simulink model "model"  (R2018b)
settings: Solver=FixedStepAuto  StartTime=0.0  StopTime=sim_time  FixedStep=Ts/10  RelTol=1e-3
StopFcn:
  | %figure;plot(true_position.Data(:,1),true_position.Data(:,2))
values from neighbouring files (symbols this model uses):
  b = ((W*a - F4*l)*cos(theta)) / (W*sin(theta)),    [blackbike_CoM.m]    (also in main.m = 1.15)
  bike_params = [g h b a lambda m]    [main.m]
  D_balancing = kd_vec(i)    [bike_linear_analysis_balancing.m]    (also in main.m = 0.01)
  D_heading = 0.01    [main.m]
  D_lateral = 0.01    [main.m]
  delay_steering = 4    [main.m]
  den_tf_steering = [1 50]    [main.m]
  g = 9.81    [main.m]
  heading_control = 0    [main.m]
  I_balancing = 0    [main.m]
  I_heading = -0.01    [main.m]
  I_lateral = 0    [main.m]
  IMU_height = 0.215    [main.m]
  initial_roll = deg2rad(2)    [main.m]
  initial_rollrate = deg2rad(1)    [main.m]
  initial_x = 0    [main.m]
  initial_y = 0    [main.m]
  lambda = deg2rad(90-24)    [main.m]
  lateral_control = 0    [main.m]
  num_tf_steering = [50]    [main.m]
  P_balancing = 1    [bike_linear_analysis_balancing.m]    (also in main.m)
  P_heading = -0.1    [main.m]
  P_lateral = -0.07    [main.m]
  path_tracking = 0    [main.m]
  path_x = path_x'    [paths.m]
  path_y = path_y'    [paths.m]
  Ts = 0.01    [main.m]
  v = 14/3.6    (= 3.88888888889)    [main.m]
undefined symbols (not defined in the file or in its folder): A, B, C, cumulative_dist_along_path, D
libraries: simulink x9, simulink_extras x7, dspsigops x2
settings Model: Creator=maximef  LastModifiedBy=maximef

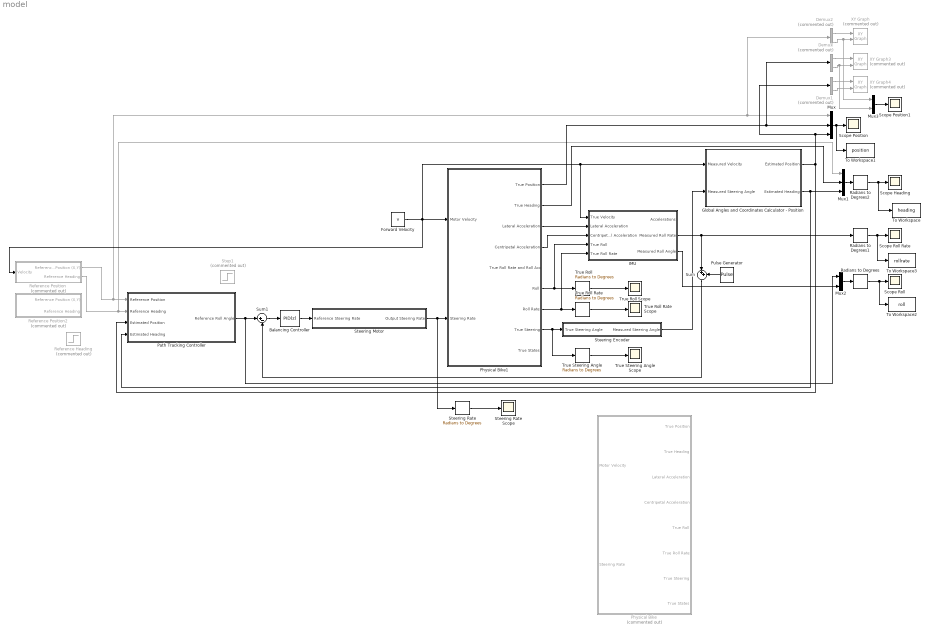
== system model ==
  Balancing Controller : simulink/Continuous/PID Controller  Controller=PID  Form=Ideal  TimeDomain=Discrete-time  SampleTime=Ts  IntegratorMethod=Trapezoidal  FilterMethod=Forward Euler  ControllerParametersSource=internal  P=P_balancing  I=I_balancing  D=D_balancing  UseFilter=off  N=5  TunerSelectOption=Transfer Function Based (PID Tuner App)  InitialConditionSource=internal  InitialConditionForIntegrator=0  InitialConditionForFilter=0  DifferentiatorICPrevScaledInput=0  ExternalReset=none  TrackingMode=off  Kt=1  LimitOutput=off  UpperSaturationLimit=inf  LowerSaturationLimit=-inf  LinearizeAsGain=on  AntiWindupMode=none  Kb=1  POutMin=[]  POutMax=[]  IOutMin=[]  IOutMax=[]  DOutMin=[]  DOutMax=[]  NOutMin=[]  NOutMax=[]  SumOutMin=[]  SumOutMax=[]  SaturationOutMin=[]  SaturationOutMax=[]  PParamMin=[]  PParamMax=[]  IParamMin=[]  IParamMax=[]  DParamMin=[]  DParamMax=[]  NParamMin=[]  NParamMax=[]  KbParamMin=[]  KbParamMax=[]  KtParamMin=[]  KtParamMax=[]  KbOutMin=[]  KbOutMax=[]  KtOutMin=[]  KtOutMax=[]  IntegratorOutMin=[]  IntegratorOutMax=[]  FilterOutMin=[]  FilterOutMax=[]  SumI1OutMin=[]  SumI1OutMax=[]  SumI2OutMin=[]  SumI2OutMax=[]  SumI3OutMin=[]  SumI3OutMax=[]  SumI4OutMin=[]  SumI4OutMax=[]  SumDOutMin=[]  SumDOutMax=[]  DifferentiatorOutMin=[]  DifferentiatorOutMax=[]  FilterDiffOutCoefMin=[]  FilterDiffOutCoefMax=[]  ReciprocalOutMin=[]  ReciprocalOutMax=[]  SumDenOutMin=[]  SumDenOutMax=[]  SumNumOutMin=[]  SumNumOutMax=[]  DivideOutMin=[]  DivideOutMax=[]  IntegratorContinuousStateAttributes=''  IntegratorStateMustResolveToSignalObject=off  IntegratorRTWStateStorageClass=Auto  FilterContinuousStateAttributes=''  FilterStateMustResolveToSignalObject=off  FilterRTWStateStorageClass=Auto  ParallelPVariant=Passthrough  IdealPVariant=InternalParameters  IVariant=InternalParameters  DVariant=InternalParameters  IntegratorVariant=Discrete  SatVariant=Disabled  AWVariant=Passthrough  PCopyVariant=Disabled  TRVariant=Disabled  FdbkBlocksVariant=Forward  IdealPFdbkVariant=Disabled  SatFdbkVariant=Disabled  DerivativeFilterVariant=Differentiator  NVariant=Passthrough  NCopyVariant=Disabled_SignalSpec  FilterICVariant=InternalICsDifferentiator  IntegratorICVariant=InternalICs  ExternalResetVariant=Disabled  TRSumVariant=Passthrough  SumFdbkVariant=Disabled  SumVariant=Sum_PID
  Demux : Demux  Commented=on  Outputs=2
  Demux1 : Demux  Commented=on  Outputs=2
  Demux2 : Demux  Commented=on  Outputs=2
  Forward Velocity : Constant  Value=v
  Global Angles and Coordinates Calculator - Position : Subsystem  SystemSampleTime=Ts
  IMU : Subsystem  TreatAsAtomicUnit=on
  Mux : Mux  Inputs=3
  Mux1 : Mux  Inputs=3
  Mux2 : Mux  Inputs=2
  Mux3 : Mux  Inputs=2
  Path Tracking Controller : Subsystem
  Physical Bike : Subsystem  Commented=on
  Physical Bike1 : Subsystem
  Pulse Generator : DiscretePulseGenerator  PulseType=Time based  Amplitude=deg2rad(1)  Period=10  PulseWidth=10
  Radians to Degrees : simulink_extras/Transformations/Radians to Degrees
  Radians to Degrees1 : simulink_extras/Transformations/Radians to Degrees
  Radians to Degrees2 : simulink_extras/Transformations/Radians to Degrees
  Reference Heading : Step  Commented=on  SampleTime=0
  Reference Position : Subsystem  Commented=on
  Reference Position2 : Subsystem  Commented=on
  Scope Heading : Scope
  Scope Position : Scope
  Scope Position1 : Scope
  Scope Roll : Scope
  Scope Roll Rate : Scope
  Steering Encoder : Subsystem  TreatAsAtomicUnit=on  SystemSampleTime=Ts
  Steering Motor : Subsystem
  Steering Rate : simulink_extras/Transformations/Radians to Degrees
  Steering Rate Scope : Scope
  Step1 : Step  Commented=on  Time=0  After=0  SampleTime=0
  Sum : Sum  Inputs=|++
  Sum1 : Sum  Inputs=|+-
  To Workspace : ToWorkspace  VariableName=heading  SaveFormat=Timeseries  SampleTime=-1
  To Workspace1 : ToWorkspace  VariableName=position  SaveFormat=Timeseries  SampleTime=-1
  To Workspace2 : ToWorkspace  VariableName=roll  SaveFormat=Timeseries  SampleTime=-1
  To Workspace3 : ToWorkspace  VariableName=rollrate  SaveFormat=Timeseries  SampleTime=-1
  True Roll : simulink_extras/Transformations/Radians to Degrees
  True Roll Rate : simulink_extras/Transformations/Radians to Degrees
  True Roll Rate Scope : Scope
  True Roll Scope : Scope
  True Steering Angle : simulink_extras/Transformations/Radians to Degrees
  True Steering Angle Scope : Scope
  XY Graph : simulink/Sinks/XY Graph  Commented=on  xmin=-10  xmax=100  ymin=-1  ymax=1  st=-1
  XY Graph3 : simulink/Sinks/XY Graph  Commented=on  xmin=-50  xmax=50  ymin=-50  ymax=50  st=-1
  XY Graph4 : simulink/Sinks/XY Graph  Commented=on  xmin=-50  xmax=50  ymin=-50  ymax=50  st=-1
  wires:
  True Roll Rate/1 -> True Roll Rate Scope/1
  True Steering Angle/1 -> True Steering Angle Scope/1
  True Roll/1 -> True Roll Scope/1
  Physical Bike1/8(True Steering) -> True Steering Angle/1, Steering Encoder/1(True Steering Angle)
  Physical Bike1/7(Roll Rate) -> IMU/5(True Roll Rate), True Roll Rate/1
  Sum1/1 -> Balancing Controller/1
  Reference Position/1(Reference Position (X,Y)) -> Demux2/1, Mux/1, Path Tracking Controller/1(Reference Position)
  Reference Position/2(Reference Heading) -> Mux1/1, Path Tracking Controller/2(Reference Heading)
  Physical Bike1/6(Roll) -> IMU/4(True Roll), True Roll/1
  Physical Bike1/2(True Heading) -> Mux1/2
  Physical Bike1/4(Centripetal Acceleration) -> IMU/3(Centripetal Acceleration)
  Forward Velocity/1 -> Reference Position/1(Velocity), Physical Bike1/1(Motor Velocity), IMU/1(True Velocity), Global Angles and Coordinates Calculator - Position/1(Measured Velocity)
  Steering Encoder/1(Measured Steering Angle) -> Global Angles and Coordinates Calculator - Position/2(Measured Steering Angle)
  Global Angles and Coordinates Calculator - Position/1(Estimated Position) -> Mux/3, Demux1/1, Path Tracking Controller/3(Estimated Position)
  Global Angles and Coordinates Calculator - Position/2(Estimated Heading) -> Path Tracking Controller/4(Estimated Heading), Mux1/3
  Mux/1 -> To Workspace1/1, Scope Position/1
  Physical Bike1/1(True Position) -> Demux/1, Mux/2
  Mux1/1 -> Radians to Degrees2/1
  IMU/3(Measured Roll Angle) -> Mux2/2
  Mux2/1 -> Radians to Degrees/1
  Path Tracking Controller/1(Reference Roll Angle) -> Sum1/1, Mux2/1
  IMU/2(Measured Roll Rate) -> Sum/1, Radians to Degrees1/1
  Radians to Degrees/1 -> To Workspace2/1, Scope Roll/1
  Radians to Degrees1/1 -> To Workspace3/1, Scope Roll Rate/1
  Radians to Degrees2/1 -> To Workspace/1, Scope Heading/1
  Demux2/1 -> XY Graph/1
  Demux/1 -> XY Graph3/1
  Demux2/2 -> Mux3/1, XY Graph/2
  Demux/2 -> Mux3/2, XY Graph3/2
  Demux1/2 -> XY Graph4/2
  Demux1/1 -> XY Graph4/1
  Mux3/1 -> Scope Position1/1
  Physical Bike1/3(Lateral Acceleration) -> IMU/2(Lateral Acceleration)
  Steering Rate/1 -> Steering Rate Scope/1
  Sum/1 -> Sum1/2
  Balancing Controller/1 -> Steering Motor/1(Reference Steering Rate)
  Steering Motor/1(Output Steering Rate) -> Physical Bike1/2(Steering Rate), Steering Rate/1
  Pulse Generator/1 -> Sum/2

== system model/Global Angles and Coordinates Calculator - Position ==
  Measured Velocity : Inport
  Measured Steering Angle : Inport  Port=2
  Gain1 : Gain  Gain=sin(lambda)
  Measured Bike Angles to Global Angles : Subsystem
  Measured Global Angles to Global Coordinates : Subsystem
  Sum : Sum  Inputs=++|
  Estimated Position : Outport
  Estimated Heading : Outport  Port=2
  wires:
  Measured Bike Angles to Global Angles/1(Psi) -> Sum/2, Measured Global Angles to Global Coordinates/2(Psi)
  Gain1/1 -> Measured Bike Angles to Global Angles/2(Measured Steering Angle)
  Sum/1 -> Estimated Heading/1
  Measured Bike Angles to Global Angles/2(Beta) -> Sum/1, Measured Global Angles to Global Coordinates/3(Beta)
  Measured Global Angles to Global Coordinates/1("Position (X, Y)") -> Estimated Position/1
  Measured Velocity/1 -> Measured Global Angles to Global Coordinates/1(Velocity), Measured Bike Angles to Global Angles/1(Velocity)
  Measured Steering Angle/1 -> Gain1/1

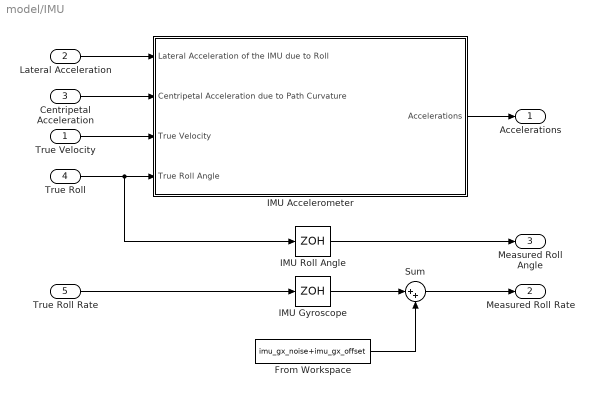
== system model/IMU ==
  True Velocity : Inport
  Lateral Acceleration : Inport  Port=2
  Centripetal Acceleration : Inport  Port=3
  True Roll : Inport  Port=4
  True Roll Rate : Inport  Port=5
  From Workspace : FromWorkspace  VariableName=imu_gx_noise+imu_gx_offset  SampleTime=0
  IMU Accelerometer : Subsystem
  IMU Gyroscope : ZeroOrderHold  SampleTime=Ts
  IMU Roll Angle : ZeroOrderHold  SampleTime=Ts
  Sum : Sum  Inputs=|++
  Accelerations : Outport
  Measured Roll Rate : Outport  Port=2
  Measured Roll Angle : Outport  Port=3
  wires:
  True Velocity/1 -> IMU Accelerometer/3(True Velocity)
  Lateral Acceleration/1 -> IMU Accelerometer/1(Lateral Acceleration of the IMU due to Roll)
  Centripetal Acceleration/1 -> IMU Accelerometer/2(Centripetal Acceleration due to Path Curvature)
  True Roll/1 -> IMU Roll Angle/1, IMU Accelerometer/4(True Roll Angle)
  IMU Accelerometer/1(Accelerations) -> Accelerations/1
  IMU Gyroscope/1 -> Sum/1
  True Roll Rate/1 -> IMU Gyroscope/1
  IMU Roll Angle/1 -> Measured Roll Angle/1
  Sum/1 -> Measured Roll Rate/1
  From Workspace/1 -> Sum/2

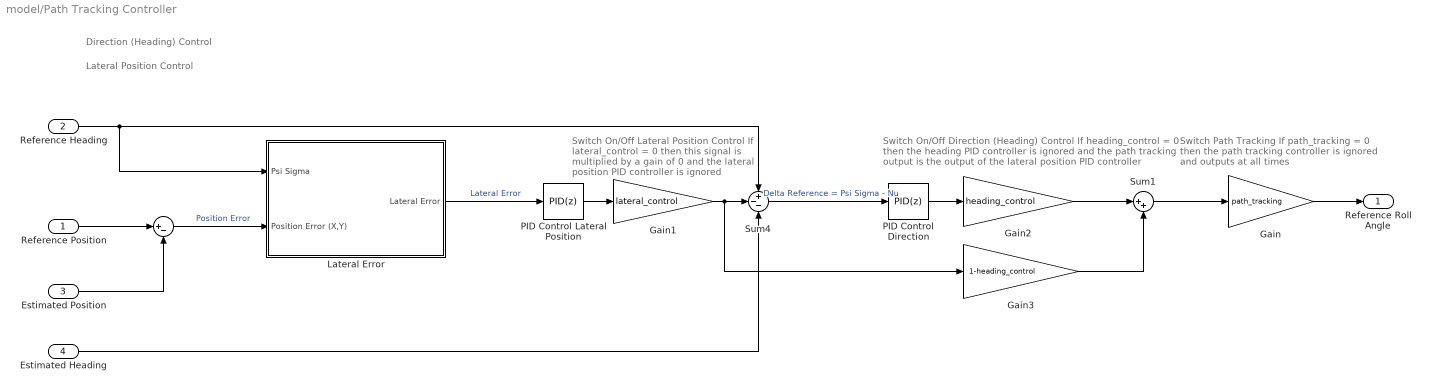
== system model/Path Tracking Controller ==
  note: Direction (Heading) Control
  note: Lateral Position Control
  note: Switch On/Off Lateral Position Control
      | If lateral_control = 0 then this signal
      | is multiplied by a gain of 0 and the
      | lateral position PID controller is ignored
  note: Switch Path Tracking
      | If path_tracking = 0 then the path tracking controller
      | is ignored and outputs at all times
  note: Switch On/Off Direction (Heading) Control
      | If heading_control = 0 then the heading PID controller is ignored
      | and the path tracking output is the output of the lateral position PID controller
  Reference Position : Inport
  Reference Heading : Inport  Port=2
  Estimated Position : Inport  Port=3
  Estimated Heading : Inport  Port=4
  " " : Sum  Inputs=|+-
  Gain : Gain  Gain=path_tracking
  Gain1 : Gain  Gain=lateral_control
  Gain2 : Gain  Gain=heading_control
  Gain3 : Gain  Gain=1-heading_control
  Lateral Error : Subsystem  SystemSampleTime=Ts
  PID Control Lateral Position : simulink/Continuous/PID Controller  Controller=PID  Form=Parallel  TimeDomain=Discrete-time  SampleTime=Ts  IntegratorMethod=Forward Euler  FilterMethod=Forward Euler  ControllerParametersSource=internal  P=P_lateral  I=I_lateral  D=D_lateral  UseFilter=on  N=100  TunerSelectOption=Transfer Function Based (PID Tuner App)  InitialConditionSource=internal  InitialConditionForIntegrator=0  InitialConditionForFilter=0  DifferentiatorICPrevScaledInput=0  ExternalReset=none  TrackingMode=off  Kt=1  LimitOutput=off  UpperSaturationLimit=inf  LowerSaturationLimit=-inf  LinearizeAsGain=on  AntiWindupMode=none  Kb=1  POutMin=[]  POutMax=[]  IOutMin=[]  IOutMax=[]  DOutMin=[]  DOutMax=[]  NOutMin=[]  NOutMax=[]  SumOutMin=[]  SumOutMax=[]  SaturationOutMin=[]  SaturationOutMax=[]  PParamMin=[]  PParamMax=[]  IParamMin=[]  IParamMax=[]  DParamMin=[]  DParamMax=[]  NParamMin=[]  NParamMax=[]  KbParamMin=[]  KbParamMax=[]  KtParamMin=[]  KtParamMax=[]  KbOutMin=[]  KbOutMax=[]  KtOutMin=[]  KtOutMax=[]  IntegratorOutMin=[]  IntegratorOutMax=[]  FilterOutMin=[]  FilterOutMax=[]  SumI1OutMin=[]  SumI1OutMax=[]  SumI2OutMin=[]  SumI2OutMax=[]  SumI3OutMin=[]  SumI3OutMax=[]  SumI4OutMin=[]  SumI4OutMax=[]  SumDOutMin=[]  SumDOutMax=[]  DifferentiatorOutMin=[]  DifferentiatorOutMax=[]  FilterDiffOutCoefMin=[]  FilterDiffOutCoefMax=[]  ReciprocalOutMin=[]  ReciprocalOutMax=[]  SumDenOutMin=[]  SumDenOutMax=[]  SumNumOutMin=[]  SumNumOutMax=[]  DivideOutMin=[]  DivideOutMax=[]  IntegratorContinuousStateAttributes=''  IntegratorStateMustResolveToSignalObject=off  IntegratorRTWStateStorageClass=Auto  FilterContinuousStateAttributes=''  FilterStateMustResolveToSignalObject=off  FilterRTWStateStorageClass=Auto  ParallelPVariant=InternalParameters  IdealPVariant=Disabled  IVariant=InternalParameters  DVariant=InternalParameters  IntegratorVariant=Discrete  SatVariant=Disabled  AWVariant=Passthrough  PCopyVariant=Disabled  TRVariant=Disabled  FdbkBlocksVariant=Forward  IdealPFdbkVariant=Disabled  SatFdbkVariant=Disabled  DerivativeFilterVariant=ForwardEulerFilter  NVariant=InternalParameters  NCopyVariant=Disabled  FilterICVariant=InternalICsFilter  IntegratorICVariant=InternalICs  ExternalResetVariant=Disabled  TRSumVariant=Passthrough  SumFdbkVariant=Disabled  SumVariant=Sum_PID
  PID Control Direction : simulink/Continuous/PID Controller  Controller=PID  Form=Parallel  TimeDomain=Discrete-time  SampleTime=Ts  IntegratorMethod=Forward Euler  FilterMethod=Forward Euler  ControllerParametersSource=internal  P=P_heading  I=I_heading  D=D_heading  UseFilter=on  N=100  TunerSelectOption=Transfer Function Based (PID Tuner App)  InitialConditionSource=internal  InitialConditionForIntegrator=0  InitialConditionForFilter=0  DifferentiatorICPrevScaledInput=0  ExternalReset=none  TrackingMode=off  Kt=1  LimitOutput=off  UpperSaturationLimit=inf  LowerSaturationLimit=-inf  LinearizeAsGain=on  AntiWindupMode=none  Kb=1  POutMin=[]  POutMax=[]  IOutMin=[]  IOutMax=[]  DOutMin=[]  DOutMax=[]  NOutMin=[]  NOutMax=[]  SumOutMin=[]  SumOutMax=[]  SaturationOutMin=[]  SaturationOutMax=[]  PParamMin=[]  PParamMax=[]  IParamMin=[]  IParamMax=[]  DParamMin=[]  DParamMax=[]  NParamMin=[]  NParamMax=[]  KbParamMin=[]  KbParamMax=[]  KtParamMin=[]  KtParamMax=[]  KbOutMin=[]  KbOutMax=[]  KtOutMin=[]  KtOutMax=[]  IntegratorOutMin=[]  IntegratorOutMax=[]  FilterOutMin=[]  FilterOutMax=[]  SumI1OutMin=[]  SumI1OutMax=[]  SumI2OutMin=[]  SumI2OutMax=[]  SumI3OutMin=[]  SumI3OutMax=[]  SumI4OutMin=[]  SumI4OutMax=[]  SumDOutMin=[]  SumDOutMax=[]  DifferentiatorOutMin=[]  DifferentiatorOutMax=[]  FilterDiffOutCoefMin=[]  FilterDiffOutCoefMax=[]  ReciprocalOutMin=[]  ReciprocalOutMax=[]  SumDenOutMin=[]  SumDenOutMax=[]  SumNumOutMin=[]  SumNumOutMax=[]  DivideOutMin=[]  DivideOutMax=[]  IntegratorContinuousStateAttributes=''  IntegratorStateMustResolveToSignalObject=off  IntegratorRTWStateStorageClass=Auto  FilterContinuousStateAttributes=''  FilterStateMustResolveToSignalObject=off  FilterRTWStateStorageClass=Auto  ParallelPVariant=InternalParameters  IdealPVariant=Disabled  IVariant=InternalParameters  DVariant=InternalParameters  IntegratorVariant=Discrete  SatVariant=Disabled  AWVariant=Passthrough  PCopyVariant=Disabled  TRVariant=Disabled  FdbkBlocksVariant=Forward  IdealPFdbkVariant=Disabled  SatFdbkVariant=Disabled  DerivativeFilterVariant=ForwardEulerFilter  NVariant=InternalParameters  NCopyVariant=Disabled  FilterICVariant=InternalICsFilter  IntegratorICVariant=InternalICs  ExternalResetVariant=Disabled  TRSumVariant=Passthrough  SumFdbkVariant=Disabled  SumVariant=Sum_PID
  Sum1 : Sum  Inputs=|++
  Sum4 : Sum  Inputs=+--
  Reference Roll Angle : Outport
  wires:
  Lateral Error/1(Lateral Error) -> PID Control Lateral Position/1  "Lateral Error"
  Estimated Position/1 -> " "/2
  " "/1 -> Lateral Error/2(Position Error (X,Y))  "Position Error"
  Sum4/1 -> PID Control Direction/1  "Delta Reference = Psi Sigma - Nu"
  Estimated Heading/1 -> Sum4/3
  Gain1/1 -> Sum4/2, Gain3/1
  PID Control Lateral Position/1 -> Gain1/1
  Reference Heading/1 -> Sum4/1, Lateral Error/1(Psi Sigma)
  Reference Position/1 -> " "/1
  Gain2/1 -> Sum1/1
  Gain3/1 -> Sum1/2
  Sum1/1 -> Gain/1
  Gain/1 -> Reference Roll Angle/1
  PID Control Direction/1 -> Gain2/1

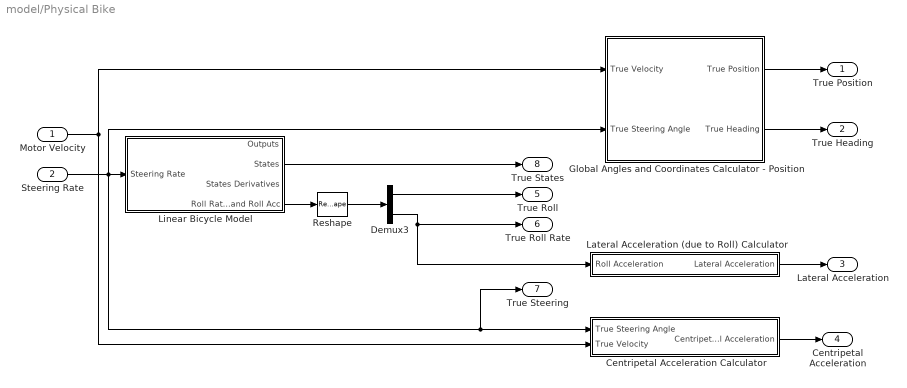
== system model/Physical Bike ==
  Motor Velocity : Inport
  Steering Rate : Inport  Port=2
  Centripetal Acceleration Calculator : Subsystem
  Demux3 : Demux  Outputs=2
  Global Angles and Coordinates Calculator - Position : Subsystem  SystemSampleTime=Ts
  Lateral Acceleration (due to Roll) Calculator : Subsystem
  Linear Bicycle Model : Subsystem
  Reshape : Reshape
  True Position : Outport
  True Heading : Outport  Port=2
  Lateral Acceleration : Outport  Port=3
  Centripetal Acceleration : Outport  Port=4
  True Roll : Outport  Port=5
  True Roll Rate : Outport  Port=6
  True Steering : Outport  Port=7
  True States : Outport  Port=8
  wires:
  Steering Rate/1 -> Global Angles and Coordinates Calculator - Position/2(True Steering Angle), True Steering/1, Centripetal Acceleration Calculator/1(True Steering Angle), Linear Bicycle Model/1(Steering Rate)
  Centripetal Acceleration Calculator/1(Centripetal Acceleration) -> Centripetal Acceleration/1
  Demux3/2 -> True Roll Rate/1, Lateral Acceleration (due to Roll) Calculator/1(Roll Acceleration)
  Lateral Acceleration (due to Roll) Calculator/1(Lateral Acceleration) -> Lateral Acceleration/1
  Linear Bicycle Model/2(States) -> True States/1
  Reshape/1 -> Demux3/1
  Linear Bicycle Model/4(Roll Rate and Roll Acc) -> Reshape/1
  Motor Velocity/1 -> Centripetal Acceleration Calculator/2(True Velocity), Global Angles and Coordinates Calculator - Position/1(True Velocity)
  Global Angles and Coordinates Calculator - Position/1(True Position) -> True Position/1
  Global Angles and Coordinates Calculator - Position/2(True Heading) -> True Heading/1
  Demux3/1 -> True Roll/1

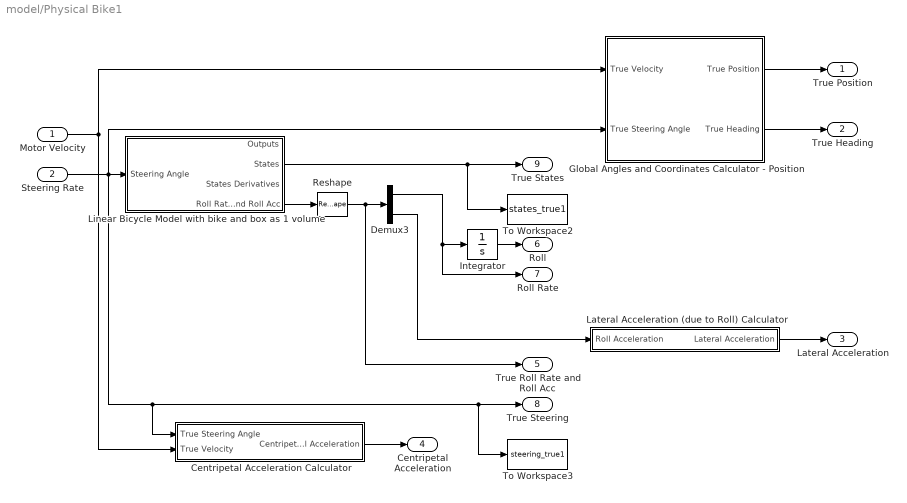
== system model/Physical Bike1 ==
  Motor Velocity : Inport
  Steering Rate : Inport  Port=2
  Centripetal Acceleration Calculator : Subsystem
  Demux3 : Demux  Outputs=2
  Global Angles and Coordinates Calculator - Position : Subsystem  SystemSampleTime=Ts
  Integrator : Integrator  InitialCondition=initial_roll
  Lateral Acceleration (due to Roll) Calculator : Subsystem
  Linear Bicycle Model with bike and box as 1 volume : Subsystem
  Reshape : Reshape
  To Workspace2 : ToWorkspace  VariableName=states_true1  SaveFormat=Timeseries  SampleTime=-1
  To Workspace3 : ToWorkspace  VariableName=steering_true1  SaveFormat=Timeseries  SampleTime=-1
  True Position : Outport
  True Heading : Outport  Port=2
  Lateral Acceleration : Outport  Port=3
  Centripetal Acceleration : Outport  Port=4
  True Roll Rate and Roll Acc : Outport  Port=5
  Roll : Outport  Port=6
  Roll Rate : Outport  Port=7
  True Steering : Outport  Port=8
  True States : Outport  Port=9
  wires:
  Steering Rate/1 -> Global Angles and Coordinates Calculator - Position/2(True Steering Angle), To Workspace3/1, True Steering/1, Centripetal Acceleration Calculator/1(True Steering Angle), Linear Bicycle Model with bike and box as 1 volume/1(Steering Angle)
  Centripetal Acceleration Calculator/1(Centripetal Acceleration) -> Centripetal Acceleration/1
  Demux3/2 -> Lateral Acceleration (due to Roll) Calculator/1(Roll Acceleration)
  Lateral Acceleration (due to Roll) Calculator/1(Lateral Acceleration) -> Lateral Acceleration/1
  Linear Bicycle Model with bike and box as 1 volume/2(States) -> To Workspace2/1, True States/1
  Demux3/1 -> Integrator/1, Roll Rate/1
  Reshape/1 -> True Roll Rate and Roll Acc/1, Demux3/1
  Linear Bicycle Model with bike and box as 1 volume/4(Roll Rate and Roll Acc) -> Reshape/1
  Motor Velocity/1 -> Centripetal Acceleration Calculator/2(True Velocity), Global Angles and Coordinates Calculator - Position/1(True Velocity)
  Global Angles and Coordinates Calculator - Position/1(True Position) -> True Position/1
  Global Angles and Coordinates Calculator - Position/2(True Heading) -> True Heading/1
  Integrator/1 -> Roll/1

== system model/Reference Position ==
  Velocity : Inport
  Integrator2 : Integrator
  Mux : Mux  Inputs=2
  Reference Position and Angle Selector : Subsystem
  Reference Position (X,Y) : Outport
  Reference Heading : Outport  Port=2
  wires:
  Reference Position and Angle Selector/3(psi_sigma) -> Reference Heading/1
  Velocity/1 -> Integrator2/1
  Reference Position and Angle Selector/2(Y_sigma) -> Mux/2
  Integrator2/1 -> Reference Position and Angle Selector/1(total travelled distance)  "total travelled distance"
  Reference Position and Angle Selector/1(X_sigma) -> Mux/1
  Mux/1 -> Reference Position (X,Y)/1

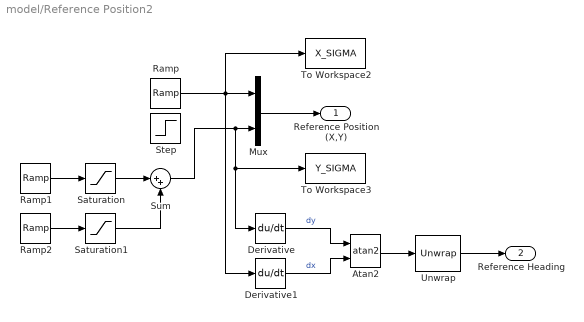
== system model/Reference Position2 ==
  Atan2 : Trigonometry  Operator=atan2
  Derivative : Derivative
  Derivative1 : Derivative
  Mux : Mux  Inputs=2
  Ramp : simulink/Sources/Ramp  slope=3  start=0  InitialOutput=0
  Ramp1 : simulink/Sources/Ramp  slope=0.01  start=5  InitialOutput=0
  Ramp2 : simulink/Sources/Ramp  slope=-0.01  start=35  InitialOutput=0
  Saturation : Saturate  UpperLimit=0.1  LowerLimit=-0.1
  Saturation1 : Saturate  UpperLimit=0.1  LowerLimit=-0.1
  Step : Step  Time=25  After=0.1  SampleTime=0
  Sum : Sum  Inputs=|++
  To Workspace2 : ToWorkspace  VariableName=X_SIGMA  SaveFormat=Timeseries  SampleTime=Ts
  To Workspace3 : ToWorkspace  VariableName=Y_SIGMA  SaveFormat=Timeseries  SampleTime=Ts
  Unwrap : dspsigops/Unwrap  tol=pi  InputProcessing=Columns as channels (frame based)  running=off
  Reference Position (X,Y) : Outport
  Reference Heading : Outport  Port=2
  wires:
  Mux/1 -> Reference Position (X,Y)/1
  Sum/1 -> Mux/2, Derivative/1, To Workspace3/1
  Ramp/1 -> Mux/1, To Workspace2/1, Derivative1/1
  Derivative1/1 -> Atan2/2  "dx"
  Atan2/1 -> Unwrap/1
  Unwrap/1 -> Reference Heading/1
  Derivative/1 -> Atan2/1  "dy"
  Ramp1/1 -> Saturation/1
  Saturation/1 -> Sum/1
  Saturation1/1 -> Sum/2
  Ramp2/1 -> Saturation1/1

== system model/Steering Encoder ==
  True Steering Angle : Inport
  Zero-Order Hold : ZeroOrderHold  SampleTime=Ts
  Measured Steering Angle : Outport
  wires:
  True Steering Angle/1 -> Zero-Order Hold/1
  Zero-Order Hold/1 -> Measured Steering Angle/1

== system model/Steering Motor ==
  Reference Steering Rate : Inport
  Delay : Delay  DelayLength=delay_steering
  Steering motor transfer function Steering Rate reference to Steering Rate : TransferFcn  Numerator=[num_tf_steering]  Denominator=[den_tf_steering]
  Output Steering Rate : Outport
  wires:
  Steering motor transfer function Steering Rate reference to Steering Rate/1 -> Output Steering Rate/1  "Realised Steering Rate"
  Reference Steering Rate/1 -> Delay/1
  Delay/1 -> Steering motor transfer function Steering Rate reference to Steering Rate/1

== system model/Global Angles and Coordinates Calculator - Position/Measured Bike Angles to Global Angles ==
  Velocity : Inport
  Measured Steering Angle : Inport  Port=2
  " Bike Parameters Model " : Constant  Value=bike_params
  Integrator : Integrator
  MATLAB Function : MATLAB Function  TreatAsAtomicUnit=on
  Psi : Outport
  Beta : Outport  Port=2
  wires:
  MATLAB Function/2(beta) -> Beta/1
  MATLAB Function/1(psi_d) -> Integrator/1
  Integrator/1 -> Psi/1
  " Bike Parameters Model "/1 -> MATLAB Function/2(parameters_model)
  Measured Steering Angle/1 -> MATLAB Function/3(delta)
  Velocity/1 -> MATLAB Function/1(v)

== system model/Global Angles and Coordinates Calculator - Position/Measured Global Angles to Global Coordinates ==
  Velocity : Inport
  Psi : Inport  Port=2
  Beta : Inport  Port=3
  Integrator1 : Integrator  InitialCondition=initial_x
  Integrator2 : Integrator  InitialCondition=initial_y
  MATLAB Function1 : MATLAB Function  TreatAsAtomicUnit=on
  Mux : Mux  Inputs=2
  "Position (X, Y)" : Outport
  wires:
  MATLAB Function1/2(Ydot) -> Integrator2/1  "Ydot"
  MATLAB Function1/1(Xdot) -> Integrator1/1  "Xdot"
  Psi/1 -> MATLAB Function1/2(psi)
  Beta/1 -> MATLAB Function1/3(beta)
  Velocity/1 -> MATLAB Function1/1(v)
  Integrator2/1 -> Mux/2
  Integrator1/1 -> Mux/1
  Mux/1 -> "Position (X, Y)"/1

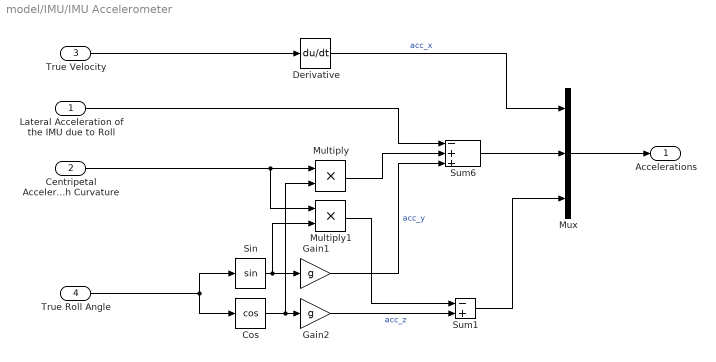
== system model/IMU/IMU Accelerometer ==
  Lateral Acceleration of the IMU due to Roll : Inport
  Centripetal Acceleration due to Path Curvature : Inport  Port=2
  True Velocity : Inport  Port=3
  True Roll Angle : Inport  Port=4
  Cos : Trigonometry  Operator=cos
  Derivative : Derivative  CoefficientInTFapproximation=-1
  Gain1 : Gain  Gain=g
  Gain2 : Gain  Gain=g
  Multiply : Product
  Multiply1 : Product
  Mux : Mux  Inputs=3
  Sin : Trigonometry
  Sum1 : Sum  Inputs=-+
  Sum6 : Sum  Inputs=-++
  Accelerations : Outport
  wires:
  Multiply/1 -> Sum6/2
  Gain1/1 -> Sum6/3  "acc_y"
  Sin/1 -> Multiply1/2, Gain1/1
  Derivative/1 -> Mux/1  "acc_x"
  Cos/1 -> Multiply/2, Gain2/1
  Gain2/1 -> Sum1/2  "acc_z"
  True Roll Angle/1 -> Sin/1, Cos/1
  True Velocity/1 -> Derivative/1
  Centripetal Acceleration due to Path Curvature/1 -> Multiply1/1, Multiply/1
  Multiply1/1 -> Sum1/1
  Sum1/1 -> Mux/3
  Mux/1 -> Accelerations/1
  Sum6/1 -> Mux/2
  Lateral Acceleration of the IMU due to Roll/1 -> Sum6/1

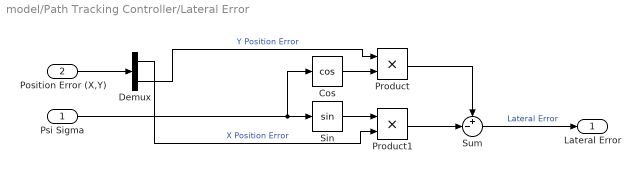
== system model/Path Tracking Controller/Lateral Error ==
  Psi Sigma : Inport
  Position Error (X,Y) : Inport  Port=2
  Cos : Trigonometry  Operator=cos
  Demux : Demux  Outputs=2
  Product : Product
  Product1 : Product
  Sin : Trigonometry
  Sum : Sum  Inputs=+-|
  Lateral Error : Outport
  wires:
  Cos/1 -> Product/2
  Sin/1 -> Product1/1
  Psi Sigma/1 -> Cos/1, Sin/1
  Product1/1 -> Sum/2
  Product/1 -> Sum/1
  Sum/1 -> Lateral Error/1  "Lateral Error"
  Demux/1 -> Product1/2  "X Position Error"
  Demux/2 -> Product/1  "Y Position Error"
  Position Error (X,Y)/1 -> Demux/1

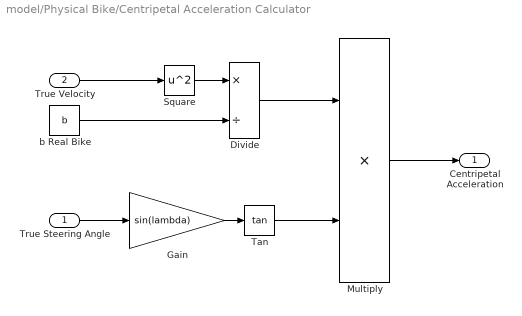
== system model/Physical Bike/Centripetal Acceleration Calculator ==
  True Steering Angle : Inport
  True Velocity : Inport  Port=2
  Divide : Product  Inputs=*/
  Gain : Gain  Gain=sin(lambda)
  Multiply : Product
  Square : Math  Operator=square  SaturateOnIntegerOverflow=on
  Tan : Trigonometry  Operator=tan
  b Real Bike : Constant  Value=b
  Centripetal Acceleration : Outport
  wires:
  True Velocity/1 -> Square/1
  Square/1 -> Divide/1
  b Real Bike/1 -> Divide/2
  True Steering Angle/1 -> Gain/1
  Divide/1 -> Multiply/1
  Tan/1 -> Multiply/2
  Multiply/1 -> Centripetal Acceleration/1
  Gain/1 -> Tan/1

== system model/Physical Bike/Global Angles and Coordinates Calculator - Position ==
  note: True Steering
      | Angle
  True Velocity : Inport
  True Steering Angle : Inport  Port=2
  Gain1 : Gain  Gain=sin(lambda)
  Measured Bike Angles to Global Angles : Subsystem
  Measured Global Angles to Global Coordinates : Subsystem
  Sum : Sum  Inputs=++|
  True Position : Outport
  True Heading : Outport  Port=2
  wires:
  Measured Bike Angles to Global Angles/1(Psi) -> Sum/2, Measured Global Angles to Global Coordinates/2(Psi)
  Gain1/1 -> Measured Bike Angles to Global Angles/2(Measured Steering Angle)
  Sum/1 -> True Heading/1
  Measured Bike Angles to Global Angles/2(Beta) -> Sum/1, Measured Global Angles to Global Coordinates/3(Beta)
  Measured Global Angles to Global Coordinates/1("Position (X, Y)") -> True Position/1
  True Velocity/1 -> Measured Global Angles to Global Coordinates/1(Velocity), Measured Bike Angles to Global Angles/1(Velocity)
  True Steering Angle/1 -> Gain1/1

== system model/Physical Bike/Lateral Acceleration (due to Roll) Calculator ==
  Roll Acceleration : Inport
  Constant3 : Constant  Value=IMU_height
  Multiply : Product
  Lateral Acceleration : Outport
  wires:
  Multiply/1 -> Lateral Acceleration/1
  Constant3/1 -> Multiply/1
  Roll Acceleration/1 -> Multiply/2

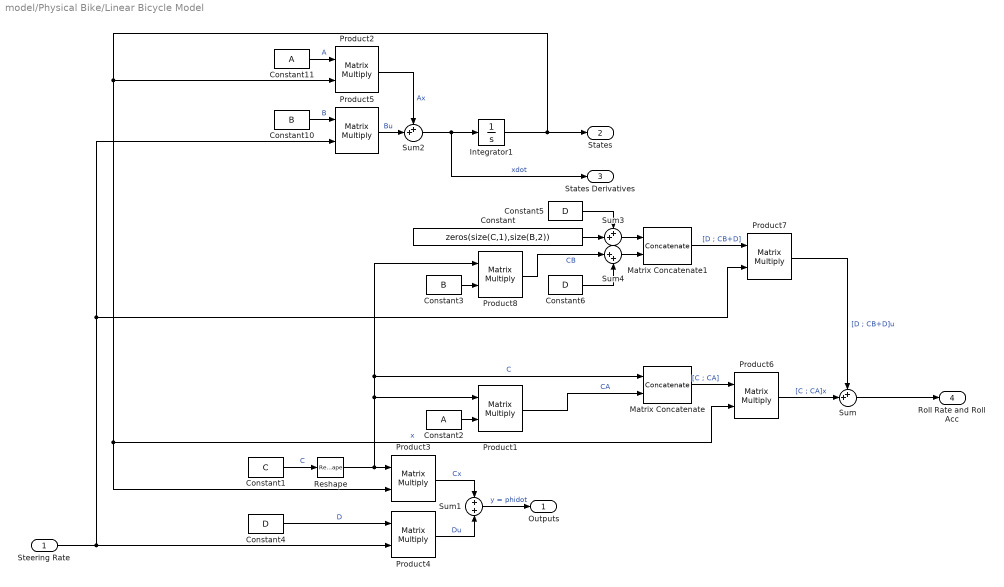
== system model/Physical Bike/Linear Bicycle Model ==
  Steering Rate : Inport
  Constant : Constant  Value=zeros(size(C,1),size(B,2))
  Constant1 : Constant  Value=C
  Constant10 : Constant  Value=B
  Constant11 : Constant  Value=A
  Constant2 : Constant  Value=A
  Constant3 : Constant  Value=B
  Constant4 : Constant  Value=D
  Constant5 : Constant  Value=D
  Constant6 : Constant  Value=D
  Integrator1 : Integrator  InitialCondition=[C ; C*A]\[initial_roll ; initial_rollrate]
  Matrix Concatenate : Concatenate  Mode=Multidimensional array
  Matrix Concatenate1 : Concatenate  Mode=Multidimensional array
  Product{1..8} (8 alike) : Product  SCDEnableBlockLinearizationSpecification=on  Multiplication=Matrix(*)
  Reshape : Reshape  OutputDimensionality=Customize  OutputDimensions=[size(C,1),size(C,2)]
  Sum : Sum  Inputs=++|
  Sum1 : Sum
  Sum2 : Sum  Inputs=++|
  Sum3 : Sum  Inputs=++|
  Sum4 : Sum  Inputs=|++
  Outputs : Outport
  States : Outport  Port=2
  States Derivatives : Outport  Port=3
  Roll Rate and Roll Acc : Outport  Port=4
  wires:
  Reshape/1 -> Product3/1, Product8/1, Matrix Concatenate/1, Product1/1  "C"
  Sum/1 -> Roll Rate and Roll Acc/1
  Constant1/1 -> Reshape/1  "C"
  Matrix Concatenate/1 -> Product6/1  "[C ; CA]"
  Product5/1 -> Sum2/2  "Bu"
  Matrix Concatenate1/1 -> Product7/1  "[D ; CB+D]"
  Constant11/1 -> Product2/1  "A"
  Constant3/1 -> Product8/2
  Product6/1 -> Sum/2  "[C ; CA]x"
  Sum2/1 -> Integrator1/1, States Derivatives/1  "xdot"
  Product2/1 -> Sum2/1  "Ax"
  Product1/1 -> Matrix Concatenate/2  "CA"
  Product8/1 -> Sum4/1  "CB"
  Integrator1/1 -> Product2/2, Product6/2, Product3/2, States/1  "x"
  Sum1/1 -> Outputs/1  "y = phidot"
  Constant2/1 -> Product1/2
  Product7/1 -> Sum/1  "[D ; CB+D]u"
  Constant10/1 -> Product5/1  "B"
  Steering Rate/1 -> Product4/2, Product5/2, Product7/2
  Product4/1 -> Sum1/2  "Du"
  Product3/1 -> Sum1/1  "Cx"
  Constant4/1 -> Product4/1  "D"
  Sum3/1 -> Matrix Concatenate1/1
  Constant/1 -> Sum3/2
  Constant5/1 -> Sum3/1
  Sum4/1 -> Matrix Concatenate1/2
  Constant6/1 -> Sum4/2

== system model/Physical Bike1/Centripetal Acceleration Calculator ==
  True Steering Angle : Inport
  True Velocity : Inport  Port=2
  Divide : Product  Inputs=*/
  Gain : Gain  Gain=sin(lambda)
  Multiply : Product
  Square : Math  Operator=square  SaturateOnIntegerOverflow=on
  Tan : Trigonometry  Operator=tan
  b Real Bike : Constant  Value=b
  Centripetal Acceleration : Outport
  wires:
  True Velocity/1 -> Square/1
  Square/1 -> Divide/1
  b Real Bike/1 -> Divide/2
  True Steering Angle/1 -> Gain/1
  Divide/1 -> Multiply/1
  Tan/1 -> Multiply/2
  Multiply/1 -> Centripetal Acceleration/1
  Gain/1 -> Tan/1

== system model/Physical Bike1/Global Angles and Coordinates Calculator - Position ==
  note: True Steering
      | Angle
  True Velocity : Inport
  True Steering Angle : Inport  Port=2
  Gain1 : Gain  Gain=sin(lambda)
  Measured Bike Angles to Global Angles : Subsystem
  Measured Global Angles to Global Coordinates : Subsystem
  Sum : Sum  Inputs=++|
  True Position : Outport
  True Heading : Outport  Port=2
  wires:
  Measured Bike Angles to Global Angles/1(Psi) -> Sum/2, Measured Global Angles to Global Coordinates/2(Psi)
  Gain1/1 -> Measured Bike Angles to Global Angles/2(Measured Steering Angle)
  Sum/1 -> True Heading/1
  Measured Bike Angles to Global Angles/2(Beta) -> Sum/1, Measured Global Angles to Global Coordinates/3(Beta)
  Measured Global Angles to Global Coordinates/1("Position (X, Y)") -> True Position/1
  True Velocity/1 -> Measured Global Angles to Global Coordinates/1(Velocity), Measured Bike Angles to Global Angles/1(Velocity)
  True Steering Angle/1 -> Gain1/1

== system model/Physical Bike1/Lateral Acceleration (due to Roll) Calculator ==
  Roll Acceleration : Inport
  Constant3 : Constant  Value=IMU_height
  Multiply : Product
  Lateral Acceleration : Outport
  wires:
  Multiply/1 -> Lateral Acceleration/1
  Constant3/1 -> Multiply/1
  Roll Acceleration/1 -> Multiply/2

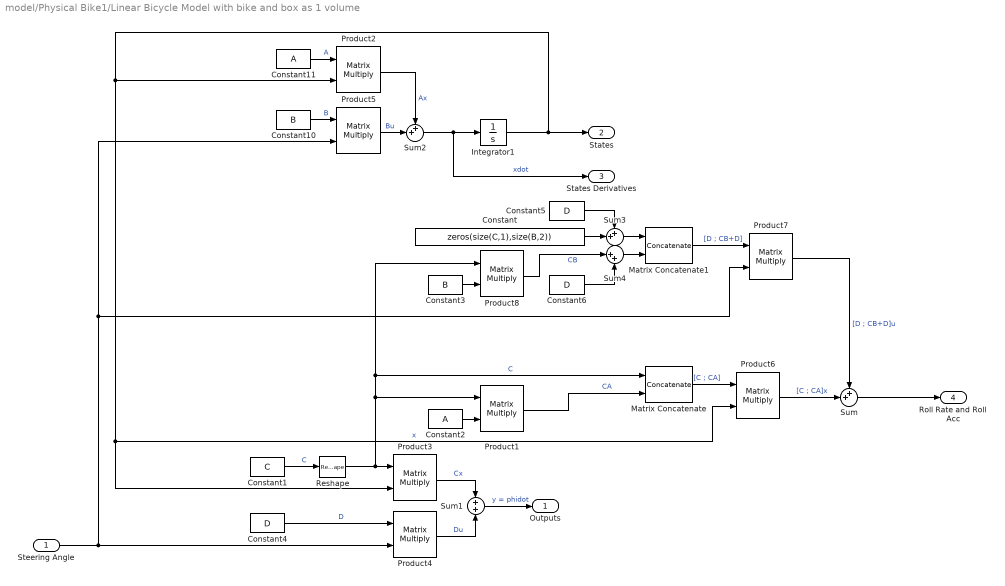
== system model/Physical Bike1/Linear Bicycle Model with bike and box as 1 volume ==
  Steering Angle : Inport
  Constant : Constant  Value=zeros(size(C,1),size(B,2))
  Constant1 : Constant  Value=C
  Constant10 : Constant  Value=B
  Constant11 : Constant  Value=A
  Constant2 : Constant  Value=A
  Constant3 : Constant  Value=B
  Constant4 : Constant  Value=D
  Constant5 : Constant  Value=D
  Constant6 : Constant  Value=D
  Integrator1 : Integrator  InitialCondition=[C ; C*A]\[initial_rollrate ; 0]
  Matrix Concatenate : Concatenate  Mode=Multidimensional array
  Matrix Concatenate1 : Concatenate  Mode=Multidimensional array
  Product{1..8} (8 alike) : Product  SCDEnableBlockLinearizationSpecification=on  Multiplication=Matrix(*)
  Reshape : Reshape  OutputDimensionality=Customize  OutputDimensions=[size(C,1),size(C,2)]
  Sum : Sum  Inputs=++|
  Sum1 : Sum
  Sum2 : Sum  Inputs=++|
  Sum3 : Sum  Inputs=++|
  Sum4 : Sum  Inputs=|++
  Outputs : Outport
  States : Outport  Port=2
  States Derivatives : Outport  Port=3
  Roll Rate and Roll Acc : Outport  Port=4
  wires:
  Reshape/1 -> Product3/1, Product8/1, Matrix Concatenate/1, Product1/1  "C"
  Sum/1 -> Roll Rate and Roll Acc/1
  Constant1/1 -> Reshape/1  "C"
  Matrix Concatenate/1 -> Product6/1  "[C ; CA]"
  Product5/1 -> Sum2/2  "Bu"
  Matrix Concatenate1/1 -> Product7/1  "[D ; CB+D]"
  Constant11/1 -> Product2/1  "A"
  Constant3/1 -> Product8/2
  Product6/1 -> Sum/2  "[C ; CA]x"
  Sum2/1 -> Integrator1/1, States Derivatives/1  "xdot"
  Product2/1 -> Sum2/1  "Ax"
  Product1/1 -> Matrix Concatenate/2  "CA"
  Product8/1 -> Sum4/1  "CB"
  Integrator1/1 -> Product2/2, Product6/2, Product3/2, States/1  "x"
  Sum1/1 -> Outputs/1  "y = phidot"
  Constant2/1 -> Product1/2
  Product7/1 -> Sum/1  "[D ; CB+D]u"
  Constant10/1 -> Product5/1  "B"
  Steering Angle/1 -> Product4/2, Product5/2, Product7/2
  Product4/1 -> Sum1/2  "Du"
  Product3/1 -> Sum1/1  "Cx"
  Constant4/1 -> Product4/1  "D"
  Sum3/1 -> Matrix Concatenate1/1
  Constant/1 -> Sum3/2
  Constant5/1 -> Sum3/1
  Sum4/1 -> Matrix Concatenate1/2
  Constant6/1 -> Sum4/2

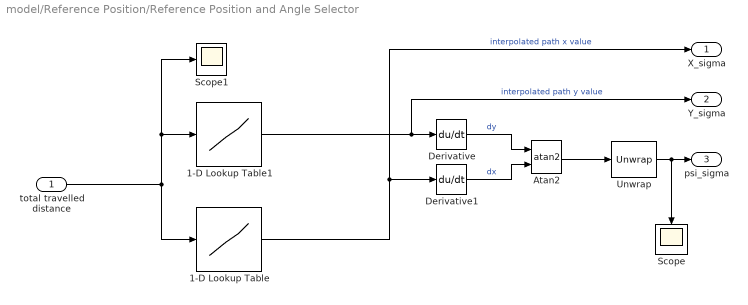
== system model/Reference Position/Reference Position and Angle Selector ==
  total travelled distance : Inport
  1-D Lookup Table : Lookup_n-D  NumberOfTableDimensions=1  BreakpointsForDimension1=cumulative_dist_along_path  Table=path_x  ExtrapMethod=Clip  DiagnosticForOutOfRangeInput=Error  InternalRulePriority=Speed  RndMeth=Simplest  InputSameDT=on
  1-D Lookup Table1 : Lookup_n-D  NumberOfTableDimensions=1  BreakpointsForDimension1=cumulative_dist_along_path  Table=path_y  ExtrapMethod=Clip  DiagnosticForOutOfRangeInput=Error  InternalRulePriority=Speed  RndMeth=Simplest  InputSameDT=on
  Atan2 : Trigonometry  Operator=atan2
  Derivative : Derivative
  Derivative1 : Derivative
  Scope : Scope
  Scope1 : Scope
  Unwrap : dspsigops/Unwrap  tol=pi  InputProcessing=Columns as channels (frame based)  running=off
  X_sigma : Outport
  Y_sigma : Outport  Port=2
  psi_sigma : Outport  Port=3
  wires:
  total travelled distance/1 -> Scope1/1, 1-D Lookup Table1/1, 1-D Lookup Table/1
  Unwrap/1 -> Scope/1, psi_sigma/1
  1-D Lookup Table/1 -> X_sigma/1, Derivative1/1  "interpolated path x value"
  Derivative1/1 -> Atan2/2  "dx"
  Derivative/1 -> Atan2/1  "dy"
  Atan2/1 -> Unwrap/1
  1-D Lookup Table1/1 -> Y_sigma/1, Derivative/1  "interpolated path y value"

== system model/Physical Bike/Global Angles and Coordinates Calculator - Position/Measured Bike Angles to Global Angles ==
  Velocity : Inport
  Measured Steering Angle : Inport  Port=2
  " Bike Parameters Model " : Constant  Value=bike_params
  Integrator : Integrator
  MATLAB Function : MATLAB Function  TreatAsAtomicUnit=on
  Psi : Outport
  Beta : Outport  Port=2
  wires:
  MATLAB Function/2(beta) -> Beta/1
  MATLAB Function/1(psi_d) -> Integrator/1
  Integrator/1 -> Psi/1
  " Bike Parameters Model "/1 -> MATLAB Function/2(bike_params)
  Measured Steering Angle/1 -> MATLAB Function/3(delta)
  Velocity/1 -> MATLAB Function/1(v)

== system model/Physical Bike/Global Angles and Coordinates Calculator - Position/Measured Global Angles to Global Coordinates ==
  Velocity : Inport
  Psi : Inport  Port=2
  Beta : Inport  Port=3
  Integrator1 : Integrator
  Integrator2 : Integrator
  MATLAB Function1 : MATLAB Function  TreatAsAtomicUnit=on
  Mux : Mux  Inputs=2
  "Position (X, Y)" : Outport
  wires:
  MATLAB Function1/2(Ydot) -> Integrator2/1  "Ydot"
  MATLAB Function1/1(Xdot) -> Integrator1/1  "Xdot"
  Psi/1 -> MATLAB Function1/2(psi)
  Beta/1 -> MATLAB Function1/3(beta)
  Velocity/1 -> MATLAB Function1/1(v)
  Integrator2/1 -> Mux/2
  Integrator1/1 -> Mux/1
  Mux/1 -> "Position (X, Y)"/1

== system model/Physical Bike1/Global Angles and Coordinates Calculator - Position/Measured Bike Angles to Global Angles ==
  Velocity : Inport
  Measured Steering Angle : Inport  Port=2
  " Bike Parameters Model " : Constant  Value=bike_params
  Integrator : Integrator
  MATLAB Function : MATLAB Function  TreatAsAtomicUnit=on
  Psi : Outport
  Beta : Outport  Port=2
  wires:
  MATLAB Function/2(beta) -> Beta/1
  MATLAB Function/1(psi_d) -> Integrator/1
  Integrator/1 -> Psi/1
  " Bike Parameters Model "/1 -> MATLAB Function/2(bike_params)
  Measured Steering Angle/1 -> MATLAB Function/3(delta)
  Velocity/1 -> MATLAB Function/1(v)

== system model/Physical Bike1/Global Angles and Coordinates Calculator - Position/Measured Global Angles to Global Coordinates ==
  Velocity : Inport
  Psi : Inport  Port=2
  Beta : Inport  Port=3
  Integrator1 : Integrator
  Integrator2 : Integrator
  MATLAB Function1 : MATLAB Function  TreatAsAtomicUnit=on
  Mux : Mux  Inputs=2
  "Position (X, Y)" : Outport
  wires:
  MATLAB Function1/2(Ydot) -> Integrator2/1  "Ydot"
  MATLAB Function1/1(Xdot) -> Integrator1/1  "Xdot"
  Psi/1 -> MATLAB Function1/2(psi)
  Beta/1 -> MATLAB Function1/3(beta)
  Velocity/1 -> MATLAB Function1/1(v)
  Integrator2/1 -> Mux/2
  Integrator1/1 -> Mux/1
  Mux/1 -> "Position (X, Y)"/1

== matlab function model/Physical Bike1/Global Angles and Coordinates Calculator - Position/Measured Bike Angles to Global Angles/MATLAB Function ==
  data: v input; bike_params input; delta input; psi_d output; beta output
function [psi_d, beta]  = fcn(v, bike_params, delta)

b = bike_params(3);
a = bike_params(4);

beta = atan((a / (b)) * tan(delta));
psi_d = (v / a) * sin(beta);

== matlab function model/Physical Bike1/Global Angles and Coordinates Calculator - Position/Measured Global Angles to Global Coordinates/MATLAB Function1 ==
  data: v input; psi input; Xdot output; beta input; Ydot output
function [Xdot, Ydot]  = fcn(v, psi, beta)

Xdot = v * cos(psi + beta);
Ydot = v * sin(psi + beta);

== matlab function model/Global Angles and Coordinates Calculator - Position/Measured Bike Angles to Global Angles/MATLAB Function ==
  data: v input; parameters_model input; delta input; psi_d output; beta output
function [psi_d, beta]  = fcn(v, parameters_model, delta)

b = parameters_model(3);
a = parameters_model(4);

beta = atan((a / (b)) * tan(delta));
psi_d = (v / a) * sin(beta);

== matlab function model/Global Angles and Coordinates Calculator - Position/Measured Global Angles to Global Coordinates/MATLAB Function1 ==
  data: v input; psi input; Xdot output; beta input; Ydot output
function [Xdot, Ydot]  = fcn(v, psi, beta)

Xdot = v * cos(psi + beta);
Ydot = v * sin(psi + beta);

== matlab function model/Physical Bike/Global Angles and Coordinates Calculator - Position/Measured Bike Angles to Global Angles/MATLAB Function ==
  data: v input; bike_params input; delta input; psi_d output; beta output
function [psi_d, beta]  = fcn(v, bike_params, delta)

b = bike_params(3);
a = bike_params(4);

beta = atan((a / (b)) * tan(delta));
psi_d = (v / a) * sin(beta);

== matlab function model/Physical Bike/Global Angles and Coordinates Calculator - Position/Measured Global Angles to Global Coordinates/MATLAB Function1 ==
  data: v input; psi input; Xdot output; beta input; Ydot output
function [Xdot, Ydot]  = fcn(v, psi, beta)

Xdot = v * cos(psi + beta);
Ydot = v * sin(psi + beta);
